simulink model "mrac_real"  (R2023b)
settings: Solver=ode45  StartTime=0.0  StopTime=700  RelTol=1e-3  EnableMultiTasking=on
undefined symbols (not defined in the file): Advantech, PCI
libraries: sldrtlib x4
settings Model: Creator=Admin  LastModifiedBy=andre
settings SolverCC: AlgebraicLoopSolver=TrustRegion
settings DataIOCC: LimitDataPoints=on  SaveFormat=Array  ReturnWorkspaceOutputs=off
settings OptimizationCC: ReuseModelBlockBuffer=off  LifeSpan=inf
settings DebuggingCC: UnconnectedInputMsg=warning  UnconnectedOutputMsg=warning  UnconnectedLineMsg=warning  SFUnexpectedBacktrackingDiag=warning  SFNoUnconditionalDefaultTransitionDiag=warning  SFExecutionAtInitializationDiag=none  ArithmeticOperatorsInVariantConditions=warning
settings HardwareCC: ProdBitPerPointer=32  ProdBitPerSizeT=32  ProdBitPerPtrDiffT=32  ProdLargestAtomicFloat=None  ProdIntDivRoundTo=Undefined  ProdEndianess=Unspecified  ProdWordSize=32  ProdHWDeviceType=32-bit Generic
settings ModelReferenceCC: PropagateSignalLabelsOutOfModel=off
settings SFSimCC: SimUseLocalCustomCode=off  CustomCodeUndefinedFunction=UseInterfaceOnly
settings RTWCC: RTWUseLocalCustomCode=off
settings CodeAppCC: StateflowObjectComments=on
settings GRTTargetCC: TargetLangStandard=C89/C90 (ANSI)
settings ConfigComp: CovMetricSettings=dw  CovSaveCumulativeToWorkspaceVar=on  CovSaveSingleToWorkspaceVar=on  CovExternalEMLEnable=off

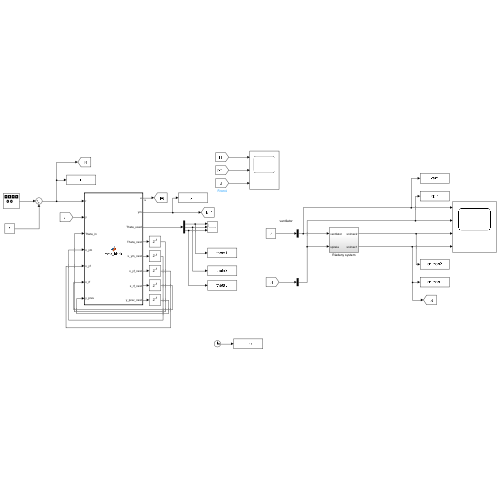
[thumbnail: Simulink's stored preview of the top-level diagram]
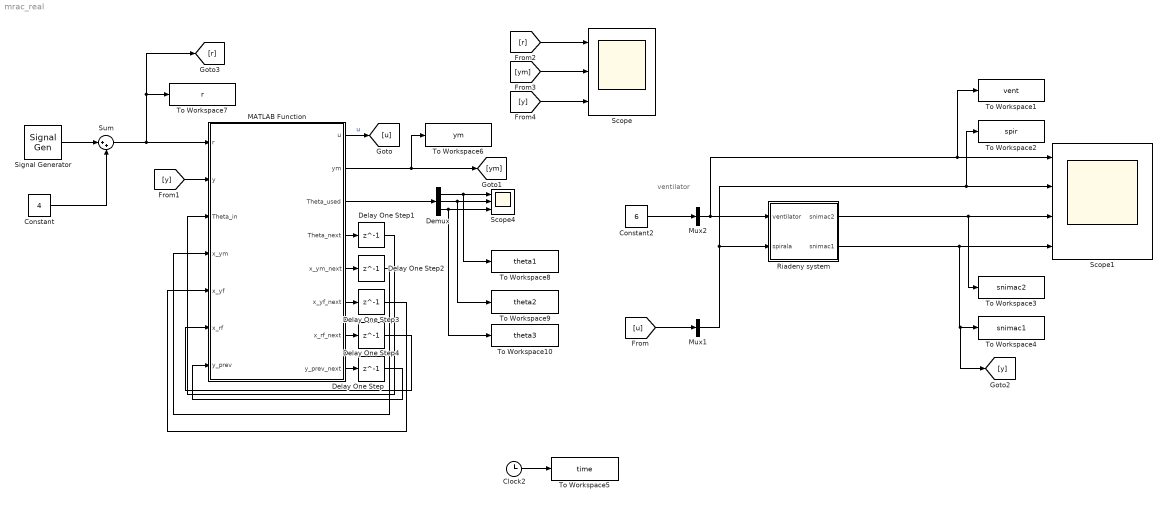
== system mrac_real ==
  note: ventilator
  Clock2 : Clock
  Constant : Constant  Value=4
  Constant2 : Constant  Value=6
  Delay One Step{,1..4} (5 alike) : Delay  DelayLength=1
  Demux : Demux  Outputs=3
  MATLAB Function : MATLAB Function  TreatAsAtomicUnit=on
  Mux1 : Mux  Inputs=1
  Mux2 : Mux  Inputs=1
  Riadeny system : Subsystem
  Scope : Scope  NumInputPorts=3
  Scope1 : Scope  NumInputPorts=4
  Scope4 : Scope  NumInputPorts=3
  Signal Generator : SignalGenerator  WaveForm=square  Amplitude=2  Frequency=1/100
  Sum : Sum  Inputs=|++
  To Workspace1 : ToWorkspace  VariableName=vent  SampleTime=0.1
      settings: Save2DSignal=2-D array (concatenate along first dimension)
  To Workspace10 : ToWorkspace  VariableName=theta3  SampleTime=0.1
      settings: Save2DSignal=2-D array (concatenate along first dimension)
  To Workspace2 : ToWorkspace  VariableName=spir  SampleTime=0.1
      settings: Save2DSignal=2-D array (concatenate along first dimension)
  To Workspace3 : ToWorkspace  VariableName=snimac2  SampleTime=0.1
      settings: Save2DSignal=2-D array (concatenate along first dimension)
  To Workspace4 : ToWorkspace  VariableName=snimac1  SampleTime=0.1
      settings: Save2DSignal=2-D array (concatenate along first dimension)
  To Workspace5 : ToWorkspace  VariableName=time  SampleTime=0.1
      settings: Save2DSignal=2-D array (concatenate along first dimension)
  To Workspace6 : ToWorkspace  VariableName=ym  SampleTime=0.1
      settings: Save2DSignal=2-D array (concatenate along first dimension)
  To Workspace7 : ToWorkspace  VariableName=r  SampleTime=0.1
      settings: Save2DSignal=2-D array (concatenate along first dimension)
  To Workspace8 : ToWorkspace  VariableName=theta1  SampleTime=0.1
      settings: Save2DSignal=2-D array (concatenate along first dimension)
  To Workspace9 : ToWorkspace  VariableName=theta2  SampleTime=0.1
      settings: Save2DSignal=2-D array (concatenate along first dimension)
  wires:
  Mux2/1 -> Riadeny system/1(ventilator), To Workspace1/1, Scope1/1
  Riadeny system/1(snimac2) -> To Workspace3/1, Scope1/3
  Riadeny system/2(snimac1) -> [y], To Workspace4/1, Scope1/4
  Mux1/1 -> Riadeny system/2(spirala), To Workspace2/1, Scope1/2
  Constant2/1 -> Mux2/1
  [u] -> Mux1/1
  Clock2/1 -> To Workspace5/1
  Delay One Step1/1 -> MATLAB Function/3(Theta_in)
  MATLAB Function/4(Theta_next) -> Delay One Step1/1
  MATLAB Function/8(y_prev_next) -> Delay One Step/1
  Demux/3 -> To Workspace10/1, Scope4/3
  MATLAB Function/3(Theta_used) -> Demux/1
  Delay One Step3/1 -> MATLAB Function/5(x_yf)
  MATLAB Function/5(x_ym_next) -> Delay One Step2/1
  Constant/1 -> Sum/2
  MATLAB Function/7(x_rf_next) -> Delay One Step4/1
  Delay One Step2/1 -> MATLAB Function/4(x_ym)
  Delay One Step/1 -> MATLAB Function/7(y_prev)
  Sum/1 -> [r], To Workspace7/1, MATLAB Function/1(r)
  Delay One Step4/1 -> MATLAB Function/6(x_rf)
  MATLAB Function/6(x_yf_next) -> Delay One Step3/1
  Demux/1 -> To Workspace8/1, Scope4/1
  Demux/2 -> To Workspace9/1, Scope4/2
  Signal Generator/1 -> Sum/1
  MATLAB Function/1(u) -> [u]  "u"
  MATLAB Function/2(ym) -> To Workspace6/1, [ym]
  [y] -> MATLAB Function/2(y)
  [r] -> Scope/1
  [ym] -> Scope/2
  [y] -> Scope/3

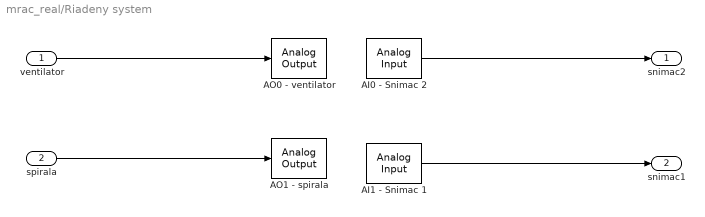
== system mrac_real/Riadeny system ==
  ventilator : Inport
  spirala : Inport  Port=2
  AI0 - Snimac 2 : sldrtlib/Analog Input  SampleTime=0.1  MaxMissedTicks=10  ShowMissedTicks=off  YieldWhenWaiting=off  DrvName=Advantech/PCI-1711  DrvAddress=4294967295  DrvOptions=zeros(1,0)  Channels=1  RangeMode=1  VoltRange=1  DataType=1
      settings: AttributesFormatString=Advantech\nPCI-1711 [auto]
  AI1 - Snimac 1 : sldrtlib/Analog Input  SampleTime=0.1  MaxMissedTicks=10  ShowMissedTicks=off  YieldWhenWaiting=off  DrvName=Advantech/PCI-1711  DrvAddress=4294967295  DrvOptions=zeros(1,0)  Channels=2  RangeMode=1  VoltRange=1  DataType=1
      settings: AttributesFormatString=Advantech\nPCI-1711 [auto]
  AO0 - ventilator : sldrtlib/Analog Output  SampleTime=0.1  MaxMissedTicks=10  ShowMissedTicks=off  YieldWhenWaiting=off  DrvName=Advantech/PCI-1711  DrvAddress=4294967295  DrvOptions=zeros(1,0)  Channels=1  RangeMode=1  VoltRange=2  InitialValue=[]  FinalValue=[]
      settings: AttributesFormatString=Advantech\nPCI-1711 [auto]
  AO1 - spirala : sldrtlib/Analog Output  SampleTime=0.1  MaxMissedTicks=10  ShowMissedTicks=off  YieldWhenWaiting=off  DrvName=Advantech/PCI-1711  DrvAddress=4294967295  DrvOptions=zeros(1,0)  Channels=2  RangeMode=1  VoltRange=2  InitialValue=[]  FinalValue=[]
      settings: AttributesFormatString=Advantech\nPCI-1711 [auto]
  snimac2 : Outport
  snimac1 : Outport  Port=2
  wires:
  ventilator/1 -> AO0 - ventilator/1
  spirala/1 -> AO1 - spirala/1
  AI1 - Snimac 1/1 -> snimac1/1
  AI0 - Snimac 2/1 -> snimac2/1

== matlab function mrac_real/MATLAB Function ==
  data: r input size=[1 1]; y input size=[1 1]; u output size=[1 1]; ym output size=[1 1]; Theta_used output size=[3 1]; Theta_in input size=[3 1]; x_ym input size=[2 1]; Theta_next output size=[3 1]; x_yf input size=[2 1]; x_rf input size=[2 1]; y_prev input size=[1 1]; x_ym_next output size=[2 1]; x_yf_next output size=[2 1]; x_rf_next output size=[2 1]; y_prev_next output size=[1 1]
function [u, ym, Theta_used, Theta_next, x_ym_next, x_yf_next, x_rf_next, y_prev_next] = mrac_block(r, y, Theta_in, x_ym, x_yf, x_rf, y_prev)

%constant_parameters
a0m = 1;
a1m = 5;
b0m = 1;

alpha1 = 0.00006;
alpha2 = 0.00001;
alpha3 = 0.00005;

sign_b0 = 1;
Ts = 0.1;

%Theta init

if all(Theta_in == 0)
    Theta = [1.309;
             8.892;
             0.165];
else
    Theta = Theta_in;
end

%Logovanie theta
Theta_used = Theta;

%Systemove matice
A = [0,    1;
     -a0m, -a1m];

b = [0;
     1];

b_ref = [0;
         b0m];

C_yf = [1, 0;
        0, 1];

C_rf = [1, 0];

C_ym = [b0m, 0];

%derivation

ydot = (y - y_prev)/Ts;

%outputs from current state

ym = C_ym * x_ym;
yf_full = C_yf * x_yf;
yf = yf_full(1);
ydot_f = yf_full(2);
rf = C_rf * x_rf;

%error

e = y - ym;

%control law

omega = [y; ydot; r];
u = Theta.' * omega;
u = max(min(u, 10), 0);

%MIT law

dTheta = -sign_b0 * e * [alpha1 * yf; 
                         alpha2 * ydot_f;     
                         alpha3 * rf];
Theta_next = Theta + dTheta * Ts;

%State updates by Euler

x_ym_next = x_ym + Ts * (A * x_ym + b * r);
x_yf_next = x_yf + Ts * (A * x_yf + b * y);
x_rf_next = x_rf + Ts * (A * x_rf + b * r);

%memory upfate for derivative

y_prev_next = y;

end
